simulink model "testsuperconst"  (R2017b)
settings: Solver=FixedStepDiscrete  StartTime=0.0  StopTime=1  RelTol=1e-3
settings Model: Creator=eruffaldi  LastModifiedBy=eruffaldi

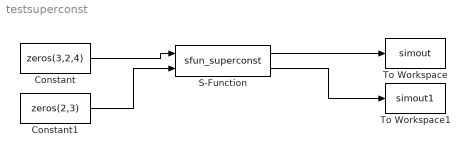
== system testsuperconst ==
  Constant : Constant  Value=zeros(3,2,4)
  Constant1 : Constant  Value=zeros(2,3)
  S-Function : S-Function  FunctionName=sfun_superconst  Parameters=1,2  SFunctionDeploymentMode=off  EnableBusSupport=off
  To Workspace : ToWorkspace  VariableName=simout  SaveFormat=Timeseries  SampleTime=-1
  To Workspace1 : ToWorkspace  VariableName=simout1  SaveFormat=Timeseries  SampleTime=-1
  wires:
  Constant/1 -> S-Function/1
  S-Function/1 -> To Workspace/1
  Constant1/1 -> S-Function/2
  S-Function/2 -> To Workspace1/1
